simulink model "commhdlQPSKTxRxLoopback"  (R2025b)
settings: Solver=FixedStepDiscrete  StartTime=0.0  StopTime=stopTime  RelTol=1e-3
PostLoadFcn:
  | hScopeConfig = get_param([gcs '/Receiver/QPSK Rx/Frequency and Time Synchronizer/Symbol Synchronizer/No HDL/QPSK Receiver Eye Diagram'],'ScopeConfiguration');
  | 
  | hScopeConfig.OpenAtSimulationStart = false;
  | hScopeConfig.Visible = false;
  | SamplesPerSymbol = 4;
  | %UpsamplesRx = 1;
  | clear hScopeConfig
InitFcn:
  | commhdlQPSKTxRxModelInit;
  | % Rate bridge: ADRV9002/Jupiter radio runs at 15.36 MHz = 2x the 7.68 MHz
  | % (4 samples/symbol @ Rsym=1.92 MHz) the QPSK Rx requires. The deployed
  | % Receiver must downsample the ADC stream by 2. UpsamplesRx=1 fed the QPSK
  | % Rx 8 sps (2x-upsampled) and broke symbol sync / the loopback bit check.
  | UpsamplesRx = 1;   %% T8 RATE FIX: rail 15.36e6 == ADC bus rate,
  | %% no ingress decimation (was 2 when the rail sat on the 7.68e6 rung)
  | UpsamplesTx = 1;
  | clear simTimingOffset;
StopFcn:
  | if exist('simTimingOffset','var')
  |   disp('Simulation completed');
  |   %QPSKTxRxVerification;
  | end
values from neighbouring files (symbols this model uses):
  Config = commhdlQPSKTxRxParameters    [commhdlQPSKTxRxModelInit.m]
  Rsym = eval(get_param(qpskFindTxInputData(gcs),'Rsym'))    [commhdlQPSKTxRxModelInit.m]
undefined symbols (not defined in the file or in its folder): Add, fsym, randsrc, RandStream, Shift
libraries: hdlsllib x143, simulink x45, dspsigops x34, dsphdlfiltering2 x6, dsphdlsigops2 x4, dsphdlmathfun2 x4, commdigbbndpm3 x4, dspmlti4 x2, commchan3 x1, commrflib2 x1, commcnvcod2 x1
(part 8 of 8)

== matlab function commhdlQPSKTxRxLoopback/TxRxComposite/CanaryFast ==
  data: x input; f2 output; f3 output; f4 output; f5 output
function [f2,f3,f4,f5] = canaryFast(x)
%#codegen
persistent r2 r3 r4 r5
if isempty(r2), r2=uint32(0); r3=uint32(0); r4=uint32(0); r5=uint32(0); end
f2=r2; f3=r3; f4=r4; f5=r5;
a = stg(x, uint32(2654435761), uint32(2166136261));
b = stg(a, uint32(2246822519), uint32(3266489917));
c = stg(b, uint32(3299170593), uint32(668265263));
d = stg(c, uint32(374761393),  uint32(2542024007));
e = stg(d, uint32(2869860233), uint32(1540483477));
r2 = b;
r3 = c;
r4 = d;
r5 = e;
end
function y = stg(x, K, C)
y = bitxor(uint32(bitand(bitshift(uint64(x) * uint64(K), -13), uint64(4294967295))), C);
end

== matlab function commhdlQPSKTxRxLoopback/TxRxComposite/CanaryRef ==
  data: x input; r2 output; r3 output; r4 output; r5 output
function [r2,r3,r4,r5] = canaryRef(x)
%#codegen
persistent m2 m3 m4 m5
if isempty(m2), m2=uint32(0); m3=uint32(0); m4=uint32(0); m5=uint32(0); end
% second halves (computed on last beat's midpoints) -- outputs match
% CanaryFast's registered outputs beat-for-beat
r2 = stg(m2, uint32(2246822519), uint32(3266489917));
c  = stg(m3, uint32(3299170593), uint32(668265263));
r3 = c;
d  = stg(stg(m4, uint32(3299170593), uint32(668265263)), uint32(374761393), uint32(2542024007));
r4 = d;
e3 = stg(stg(m5, uint32(3299170593), uint32(668265263)), uint32(374761393), uint32(2542024007));
r5 = stg(e3, uint32(2869860233), uint32(1540483477));
% first halves for NEXT beat
a = stg(x, uint32(2654435761), uint32(2166136261));
b = stg(a, uint32(2246822519), uint32(3266489917));
m2 = a;
m3 = b;
m4 = b;
m5 = b;
end
function y = stg(x, K, C)
y = bitxor(uint32(bitand(bitshift(uint64(x) * uint64(K), -13), uint64(4294967295))), C);
end

== matlab function commhdlQPSKTxRxLoopback/TxRxComposite/CanaryScore ==
  data: f2 input; y output; f3 input; f4 input; f5 input; r2 input; r3 input; r4 input; r5 input
function y = canaryScore(f2,f3,f4,f5,r2,r3,r4,r5)
%#codegen
persistent c2 c3 c4 c5 warm
if isempty(c2), c2=uint8(0); c3=uint8(0); c4=uint8(0); c5=uint8(0); warm=uint8(0); end
if warm < uint8(8)
  warm = warm + uint8(1);
else
  if f2 ~= r2 && c2 < uint8(255), c2 = c2 + uint8(1); end
  if f3 ~= r3 && c3 < uint8(255), c3 = c3 + uint8(1); end
  if f4 ~= r4 && c4 < uint8(255), c4 = c4 + uint8(1); end
  if f5 ~= r5 && c5 < uint8(255), c5 = c5 + uint8(1); end
end
y = bitor(bitor(uint32(c2), bitshift(uint32(c3),8)), ...
          bitor(bitshift(uint32(c4),16), bitshift(uint32(c5),24)));

== matlab function commhdlQPSKTxRxLoopback/Transmitter/QPSK Tx/Bit Packetizer/Data Bits FIFO/MATLAB Function1 ==
  data: wr input; full output; rd input; dataBitsPerPacket parameter
function full = fcn(wr,rd,dataBitsPerPacket)
%#codegen
     
    depth = dataBitsPerPacket*2 - 1;
    persistent count;
    if isempty(count)
        count = fi(0,0,nextpow2(depth),0,hdlfimath);
    end

    if wr
        count(:) = count + 1;
    end
    if rd
        count(:) = count - 1;
    end

    full = (count > depth);

end

== matlab function commhdlQPSKTxRxLoopback/TxRxComposite/Receiver/QPSK Rx/Frequency and Time Synchronizer/Symbol Synchronizer/Interpolation Control Shadow ==
  data: Delta input; mu output; Underflow output
function [mu,Underflow] = Interpolation_ctrl(Delta)
% Implementation of modulo-1 counter for interpolation control listed in
% Figure 8.4.19 of "Digital Communications - A Discrete-Time Approach"
% by Michael Rice. See design details in Chapter 8.4.3 of the same book.
% 
% Input:
%   Delta - Loop filter output. If loop is in lock, delta would be small
% Output:
%   Underflow - Indicator of counter underflow. This is the strobe signal
%               for downstream processing
%   mu - Difference between actual sampling instant and the optimal instant,
%        between zero and one
%#codegen

% countReg - Counter value delayed by 1 sample
% muReg - The estimated timing error normalized by half QPSK symbols

   mask = fi(1-2^(-10),1,11,10);
   
   persistent countReg underflowReg muReg;
   if isempty(countReg)
       countReg  = fi(0.125,1,11,10); %% shadow leading-beat offset compensation
       muReg = fi(0,1,11,10);
       underflowReg = false;
   end
   
   
   Underflow = underflowReg;
   mu = muReg;   
   
   
      % T8.4 anti-wedge clamp: if Delta <= -0.125 the decrementing counter
   % never underflows (strobes stop FOREVER -- Class-4 wedge / Class-1
   % episode mechanism; see tb_timing_wedge.v). Bound Delta so the
   % counter always decrements by >= 1 LSB.
   wlim = fi(127/1024,1,11,10);
   if Delta > wlim
       Delta = wlim;
   elseif Delta < -wlim
       Delta = fi(-127/1024,1,11,10);
   end
   counter = bitand(mask,countReg)-Delta-fi(0.125,1,11,10); % decrementing counter
   
   % if countReg is a nonnegative number,
   % then mod(countReg,1) equals the fractional part of countReg
   if counter < 0
       underflowReg = true;
       muReg = bitshift(bitand(mask,countReg),3);
       countReg = fi(counter+1,1,11,10);% create underflow to counter
   else
       underflowReg = false;
       countReg = fi(counter,1,11,10);
   end
   


end

== matlab function commhdlQPSKTxRxLoopback/TxRxComposite/Receiver/QPSK Rx/Frequency and Time Synchronizer/Symbol Synchronizer/ShadowScoreIC ==
  data: muP input; divBeat output; muS input; undP input; undS input; divCnt output
function [divBeat, divCnt] = shadowScoreIC(muP, muS, undP, undS)
%#codegen
persistent db dc bt mPrev
if isempty(db), db=uint32(0); dc=uint32(0); bt=uint32(0); mPrev=false; end
bt = bt + uint32(1);
m = (muP ~= muS) || (undP ~= undS);
if m && ~mPrev
  if db == uint32(0), db = bt; end
  if dc < uint32(4294967295), dc = dc + uint32(1); end
end
mPrev = m;
divBeat = db; divCnt = dc;

== matlab function commhdlQPSKTxRxLoopback/TxRxComposite/Receiver/QPSK Rx/Frequency and Time Synchronizer/Carrier Synchronizer/ShadowScoreCS ==
  data: pP input; divBeat output; pS input; iP input; iS input; divCnt output
function [divBeat, divCnt] = shadowScoreCS(pP, pS, iP, iS)
%#codegen
persistent db dc bt mPrev
if isempty(db), db=uint32(0); dc=uint32(0); bt=uint32(0); mPrev=false; end
bt = bt + uint32(1);
m = (pP ~= pS) || (iP ~= iS);
if m && ~mPrev
  if db == uint32(0), db = bt; end
  if dc < uint32(4294967295), dc = dc + uint32(1); end
end
mPrev = m;
divBeat = db; divCnt = dc;

== matlab function commhdlQPSKTxRxLoopback/TxRxComposite/Receiver/QPSK Rx/TelemetrySerializer ==
  data: ssI input fixdt(1,30,23); telI output fixdt(1,16,0); ssP input fixdt(1,30,23); ssD4 input fixdt(1,30,23); ssD6 input fixdt(1,30,23); ssD3 input fixdt(1,30,23); ssD5 input fixdt(1,30,23); ssD2 input fixdt(1,40,24); icW input uint32; csP input fixdt(1,29,29); csI input fixdt(1,39,39); csD7 input fixdt(1,13,10); csD5 input fixdt(1,13,10); csD6 input fixdt(1,29,26); csD2 input fixdt(1,29,29); csD1 input fixdt(1,29,26); csD3 input fixdt(1,39,39); agcI input fixdt(1,34,28); telQ output fixdt(1,16,0)
function [telI, telQ] = telemetrySerializer(ssI, ssP, ssD4, ssD6, ssD3, ssD5, ssD2, icW, ...
    csP, csI, csD7, csD5, csD6, csD2, csD1, csD3, agcI)
%#codegen
persistent slot img
if isempty(slot), slot = uint8(0); img = uint32(0); end
w = uint32(0);
switch slot
  case uint8(0),  w = uint32(reinterpretcast(ssI,  numerictype(0,30,0)));
  case uint8(1),  w = uint32(reinterpretcast(ssP,  numerictype(0,30,0)));
  case uint8(2),  w = uint32(reinterpretcast(ssD4, numerictype(0,30,0)));
  case uint8(3),  w = uint32(reinterpretcast(ssD6, numerictype(0,30,0)));
  case uint8(4),  w = uint32(reinterpretcast(ssD3, numerictype(0,30,0)));
  case uint8(5),  w = uint32(reinterpretcast(ssD5, numerictype(0,30,0)));
  case uint8(6),  w = uint32(bitsliceget(reinterpretcast(ssD2, numerictype(0,40,0)), 32, 1));
  case uint8(7),  w = uint32(bitsliceget(reinterpretcast(ssD2, numerictype(0,40,0)), 40, 33));
  case uint8(8),  w = icW;
  case uint8(9),  w = uint32(reinterpretcast(csP, numerictype(0,29,0)));
  case uint8(10), w = uint32(bitsliceget(reinterpretcast(csI, numerictype(0,39,0)), 32, 1));
  case uint8(11), w = uint32(bitsliceget(reinterpretcast(csI, numerictype(0,39,0)), 39, 33));
  case uint8(12), w = bitor(uint32(reinterpretcast(csD7, numerictype(0,13,0))), ...
                      bitshift(uint32(reinterpretcast(csD5, numerictype(0,13,0))), 13));
  case uint8(13), w = uint32(reinterpretcast(csD6, numerictype(0,29,0)));
  case uint8(14), w = uint32(reinterpretcast(csD2, numerictype(0,29,0)));
  case uint8(15), w = uint32(reinterpretcast(csD1, numerictype(0,29,0)));
  case uint8(16), w = uint32(bitsliceget(reinterpretcast(csD3, numerictype(0,39,0)), 32, 1));
  case uint8(17), w = uint32(bitsliceget(reinterpretcast(csD3, numerictype(0,39,0)), 39, 33));
  case uint8(18), w = uint32(bitsliceget(reinterpretcast(real(agcI), numerictype(0,34,0)), 32, 1));
  case uint8(19), w = uint32(bitsliceget(reinterpretcast(real(agcI), numerictype(0,34,0)), 34, 33));
  case uint8(20), w = uint32(bitsliceget(reinterpretcast(imag(agcI), numerictype(0,34,0)), 32, 1));
  case uint8(21), w = uint32(bitsliceget(reinterpretcast(imag(agcI), numerictype(0,34,0)), 34, 33));
  case uint8(22), w = uint32(2781216750);
  otherwise,      w = img;
end
slot = slot + uint8(1);
if slot >= uint8(24)
  slot = uint8(0);
  img = img + uint32(1);
end
telI = reinterpretcast(uint16(bitshift(w, -16)), numerictype(1,16,0));
telQ = reinterpretcast(uint16(bitand(w, uint32(65535))), numerictype(1,16,0));

== matlab function commhdlQPSKTxRxLoopback/TxRxComposite/Transmitter/Input Data/ByteBitShifter ==
  data: enable input; bit output; reset input; start input; extWord input; extWordAvail input; extWordFirst input; popToggle output
function [bit, popToggle] = byteBitShifterBlk(enable, reset, start, extWord, extWordAvail, extWordFirst)
% Block wrapper around qpskByteBitShifter (the unit-tested single source
% of truth). Persistent state only; the effective enable matches the
% Message Generator chart's active condition (enable && ~reset) so the
% shifter emits bits on exactly the generator's bit steps. pop is
% exported as a toggle (one flip per word latch OR discard) to survive
% the slow->fast rate crossing; upstream edge-detects it into a pulse.
persistent state tog
if isempty(state)
    state = qpskByteBitShifter();
    tog = false;
end
en = logical(enable) && ~logical(reset);
[bit, pop, state] = qpskByteBitShifter(state, en, logical(start), ...
    uint64(extWord), logical(extWordAvail), logical(extWordFirst));
if pop
    tog = ~tog;
end
popToggle = tog;

== matlab function commhdlQPSKTxRxLoopback/TxRxComposite/Transmitter/Input Data/FEC Tx Encoder K5/TxGateK5 ==
  data: bitIn input; infoBit output; enable input; reset input; start input; encReset output; infoValid output; beatIdx output; frameValid output; frameStart output
function [infoBit, encReset, infoValid, beatIdx, frameValid, frameStart] = fecTxGateK5(bitIn, enable, reset, start)
%#codegen
% sync-semantics (RXROOT E11c): locals in, outputs from locals, persist last.
persistent beat armed;
INFO=uint16(1084); NIN=uint16(1088); PAYLOAD=uint16(2240);
if isempty(beat), beat=uint16(0); armed=false; end
b=beat; a=armed;
infoBit=false; encReset=false; infoValid=false; beatIdx=uint16(0);
frameValid=false; frameStart=false;
en = logical(enable) && ~logical(reset);
if en
  if start, b=uint16(0); a=true; encReset=true; end
  if a
    if b < INFO
      infoBit = logical(bitIn); infoValid = true;
    elseif b < NIN
      infoBit = false;          infoValid = true;   % K-1 zero tail flush
    end
    beatIdx = b; frameValid = true; frameStart = (b==uint16(0));
    if b < PAYLOAD-uint16(1), b=b+uint16(1); else, b=uint16(0); end
  end
end
beat=b; armed=a;

== matlab function commhdlQPSKTxRxLoopback/TxRxComposite/Transmitter/Input Data/FEC Tx Encoder K5/ConvEncK5 ==
  data: infoBit input; codedPair output; encReset input; infoValid input
function codedPair = fecConvEncK5(infoBit, encReset, infoValid)
%#codegen
persistent sr;
if isempty(sr), sr = false(1,4); end
srUse = sr;
if encReset, srUse = false(1,4); end   % reset-then-advance (zero frame state)
in = logical(infoBit);
s0=in; s1=srUse(1); s2=srUse(2); s3=srUse(3); s4=srUse(4);
g0 = xor(s0, xor(s1, xor(s2, s4)));   % poly 35 oct = 11101
g1 = xor(s0, xor(s3, s4));            % poly 23 oct = 10011
codedPair = [g0; g1];
% state update: advance ONLY on infoValid, else HOLD (anti-zero-stuff gate)
if infoValid
  sr = [in, srUse(1:3)];
else
  sr = srUse;
end

== matlab function commhdlQPSKTxRxLoopback/Transmitter/QPSK Tx/Bit Packetizer/Data Bits FIFO/RAM Frame Status Indicator ==
  data: push input; out output; pop input; dataBitsPerPacket parameter
function out = fcn(push,pop,dataBitsPerPacket)

   persistent pushCount popCount frameCount;
   if isempty(pushCount)
       pushCount = fi(0,0,nextpow2(dataBitsPerPacket),0,hdlfimath);
       frameCount = fi(0,0,2,0,hdlfimath);
       popCount = fi(0,0,nextpow2(dataBitsPerPacket),0,hdlfimath);
   end
   
   if (pushCount == dataBitsPerPacket-1) && push
       frameCount(:) = frameCount + 1;
   end
   if (popCount == dataBitsPerPacket-1) && pop
       frameCount(:) = frameCount - 1;
   end

   if push
       if pushCount == dataBitsPerPacket - 1
           pushCount(:) = 0;
       else
           pushCount(:) = pushCount + 1;
       end
   end

   if pop 
       if popCount == dataBitsPerPacket - 1
           popCount(:) = 0;
       else
           popCount(:) = popCount + 1;
       end
   end

   out = frameCount;

end

== matlab function commhdlQPSKTxRxLoopback/TxRxComposite/Transmitter/Input Data/FEC Tx Encoder K5/TxInterleaveK5 ==
  data: codedPair input; dataOut output; infoValid input; beatIdx input; frameValid input; frameStart input
function dataOut = fecTxInterleaveK5(codedPair, infoValid, beatIdx, frameValid, frameStart)
%#codegen
persistent ramA ramB rdBank wptr rrow rcol;
CODED=uint16(2176); COLS=uint16(16); ROWS=uint16(136);
FILL = logical([1 1 1 1 1 1 1 1 1 0 0 0 0 0 1 1 1 1 0 1 1 1 1 1 0 0 0 1 0 1 1 1 0 0 1 1 0 0 1 0 0 0 0 0 1 0 0 1 0 1 0 0 1 1 1 0 1 1 0 1 0 0 0 1]);   % 64-bit PN9 filler (T8 fix 6bcaa62)
if isempty(ramA), ramA=false(1,2176); ramB=false(1,2176); rdBank=false; wptr=uint16(0); rrow=uint16(0); rcol=uint16(0); end
rb=rdBank; w=wptr; rr=rrow; cc=rcol;
dataOut=false;
wr0=uint16(0); wr1=uint16(0); v0=false; v1=false; doW0=false; doW1=false;
if frameValid
  if frameStart, w=uint16(0); rb=~rb; end
  % ---- READ side (previous frame, opposite bank), legacy perm r*COLS+c ----
  % divisionless read address: rr (row 0..ROWS-1) / cc (col 0..COLS-1) are
  % incremental counters, reset on beatIdx==0, advancing +1 row with col carry
  % per in-range beat -- replaces the old per-beat divide-by-ROWS. No divide.
  if beatIdx < CODED
    % precondition: bit-exactness requires a contiguous beatIdx hitting 0 once per
    % frame to re-seed the row/col counters (the old stateless per-beat address
    % arithmetic derived the address from beatIdx alone and needed no such reset).
    if beatIdx == 0, rr = uint16(0); cc = uint16(0); end
    perm = rr*COLS + cc;
    if perm < CODED
      if rb, dataOut = ramB(double(perm)+1); else, dataOut = ramA(double(perm)+1); end
    end
    rr = rr + uint16(1);
    if rr == ROWS, rr = uint16(0); cc = cc + uint16(1); end
  else
    dataOut = FILL(double(beatIdx-CODED)+1);   % PN9 filler, beats CODED..2239
  end
  % ---- WRITE side: two coded bits per encoder-advance beat ----
  if infoValid
    if w < CODED, wr0=w; v0=(codedPair(1)~=0); doW0=true; w=w+uint16(1); end
    if w < CODED, wr1=w; v1=(codedPair(2)~=0); doW1=true; w=w+uint16(1); end
  end
end
% ---- persist state last (write bank = opposite of read bank) ----
if doW0
  if rb, ramA(double(wr0)+1)=v0; else, ramB(double(wr0)+1)=v0; end
end
if doW1
  if rb, ramA(double(wr1)+1)=v1; else, ramB(double(wr1)+1)=v1; end
end
rdBank=rb; wptr=w; rrow=rr; rcol=cc;

== matlab function commhdlQPSKTxRxLoopback/TxRxComposite/ByteWordBuffer ==
  data: dataIn input; word output; validIn input; popReq input; firstIn input; avail output; readyNext output; wordFirst output
function [word, avail, readyNext, wordFirst] = byteWordBufferBlk(dataIn, validIn, popReq, firstIn)
% Block wrapper around qpskByteWordBuffer (unit-tested single source of
% truth); persistent state only. readyNext = the post-update registered
% ready; an external Delay (IC=1) turns it back into the AXIS tready.
% firstIn/wordFirst carry the in-band first-word marker alongside data.
persistent state
if isempty(state)
    state = qpskByteWordBuffer();
end
[word, avail, ~, wordFirst, state] = qpskByteWordBuffer(state, uint64(dataIn), ...
    logical(validIn), logical(popReq), logical(firstIn));
readyNext = state.readyReg;

== matlab function commhdlQPSKTxRxLoopback/TxRxComposite/ByteSerializer ==
  data: bitIn input; word output; bitValid input; start input; ready input; wordTog output; wordLast output; wordFirst output
function [word, wordTog, wordLast, wordFirst] = byteSerializerBlk(bitIn, bitValid, start, ready)
% Block wrapper around qpskByteSerializer (unit-tested single source of
% truth); persistent state only. word/wordLast are HELD stable between
% emissions; wordTog flips once per emitted word so the slow->fast rate
% crossing cannot drop or repeat it -- the 30.72M BeatGate edge-detects
% it into exactly one accepted AXIS beat. Dropped words (ready low at
% completion) do not toggle: drop means NO beat, never a stall.
% K5 kit: 16 words/frame = the first 64*16 of
% the 1084 decoded info bits; the trailing 60 are dropped by start-reset.
persistent state tog heldWord heldLast heldFirst firstNext
if isempty(state)
    state = qpskByteSerializer();
    tog = false; heldWord = uint64(0); heldLast = false;
    heldFirst = true; firstNext = true;
end
% presentation is decoupled from acceptance (ADI S2MM source style):
% the offered beat must refresh on EVERY completed word or the DMA's
% SYNC_TRANSFER_START gate can wait forever on a frozen user flag /
% accept a stale word. ready at the pin only decides acceptance, so
% the core serializer runs with ready=true and unaccepted beats are
% simply superseded.
[w, wv, wl, ~, state] = qpskByteSerializer(state, logical(bitIn), ...
    logical(bitValid), logical(start), true, uint16(16));
if wv
    heldWord = w; heldLast = logical(wl); tog = ~tog;
    heldFirst = firstNext; firstNext = logical(wl);
end
word = heldWord; wordTog = tog; wordLast = heldLast; wordFirst = heldFirst;

== matlab function commhdlQPSKTxRxLoopback/TxRxComposite/ByteRxFifo ==
  data: word input uint64; outWord output uint64; tog input boolean; wLast input boolean; wFirst input boolean; ready input boolean; valid output boolean; outLast output boolean; outFirst output boolean; ovf output uint32
function [outWord, valid, outLast, outFirst, ovf] = byteRxFifo(word, tog, wLast, wFirst, ready)
%#codegen
% 64-deep elastic FIFO: enqueue on serializer toggle edge, dequeue on
% accepted AXIS beat. Drop-newest + count on full (stall > ~19 ms).
persistent mem memFl wr rd prev ovfCnt
if isempty(wr)
    mem = zeros(64,1,'uint64'); memFl = zeros(64,1,'uint8');
    wr = uint16(0); rd = uint16(0); prev = false; ovfCnt = uint32(0);
end
if logical(tog) ~= prev
    nxt = uint16(mod(uint32(wr) + 1, 64));
    if nxt == rd
        % full: DROP OLDEST (advance rd) so the presented head converges
        % to fresh data when unconsumed -- preserves the DMA start-sync
        % contract (the old supersede semantics) while keeping 64 words
        % of elasticity for transient stalls. Never deadlocks on a
        % mid-frame stale head.
        rd = uint16(mod(uint32(rd) + 1, 64));
        ovfCnt = ovfCnt + uint32(1);
    end
    mem(uint32(wr)+1)   = uint64(word);
    memFl(uint32(wr)+1) = uint8(wLast) + uint8(2)*uint8(wFirst);
    wr = nxt;
end
prev = logical(tog);
valid = (wr ~= rd);
outWord  = mem(uint32(rd)+1);
fl = memFl(uint32(rd)+1);
outLast  = bitand(fl, uint8(1)) ~= uint8(0);
outFirst = bitand(fl, uint8(2)) ~= uint8(0);
if valid && logical(ready)
    rd = uint16(mod(uint32(rd) + 1, 64));
end
ovf = ovfCnt;

== matlab function commhdlQPSKTxRxLoopback/TxRxComposite/Receiver/QPSK Rx/Frequency and Time Synchronizer/Carrier Synchronizer/ValidCensus ==
  data: vin input boolean; cvin output uint32; vlf input boolean; vout input boolean; cvlf output uint32; cvout output uint32
function [cvin, cvlf, cvout] = validCensus(vin, vlf, vout)
%#codegen
persistent a b c
if isempty(a), a = uint32(0); b = uint32(0); c = uint32(0); end
if vin,  a = a + uint32(1); end
if vlf,  b = b + uint32(1); end
if vout, c = c + uint32(1); end
cvin = a; cvlf = b; cvout = c;

== matlab function commhdlQPSKTxRxLoopback/TxRxComposite/ByteCensus ==
  data: v input boolean; cnt output uint32
function cnt = byteCensus(v)
%%#codegen
persistent a
if isempty(a), a = uint32(0); end
if v, a = a + uint32(1); end
cnt = a;

== matlab function commhdlQPSKTxRxLoopback/TxRxComposite/Receiver/QPSK Rx/Frequency and Time Synchronizer/Preamble Detector/PdCensus ==
  data: done input boolean; w1 output uint32; succ input boolean; off input uint16; taSync input boolean; nEnt input uint8; vPop input boolean; w2 output uint32; w3 output uint32
function [w1, w2, w3] = pdCensus(done, succ, off, taSync, nEnt, vPop)
%#codegen
persistent cDone cSucc pSucc cSync cPop hiw offL
if isempty(cDone)
    cDone = uint32(0); cSucc = uint32(0); pSucc = false;
    cSync = uint32(0); cPop = uint32(0); hiw = uint8(0); offL = uint16(0);
end
if done,   cDone = cDone + uint32(1); offL = off; end
if succ && ~pSucc, cSucc = cSucc + uint32(1); end
pSucc = logical(succ);
if taSync, cSync = cSync + uint32(1); end
if vPop,   cPop  = cPop  + uint32(1); end
if nEnt > hiw, hiw = nEnt; end
w1 = bitor(bitshift(bitand(cSync, uint32(65535)), 16), bitand(cDone, uint32(65535)));
w2 = bitor(bitor(bitshift(uint32(hiw), 24), ...
     bitshift(bitand(cSucc, uint32(255)), 16)), uint32(offL));
w3 = cPop;

== matlab function commhdlQPSKTxRxLoopback/TxRxComposite/Receiver/QPSK Rx/Frequency and Time Synchronizer/Packet Controller/PcCensus ==
  data: pend input boolean; w1 output uint32; endp input boolean; startp input boolean; w2 output uint32
function [w1, w2] = pcCensus(pend, endp, startp)
%#codegen
persistent cPend pPend cEnd cStart
if isempty(cPend)
    cPend = uint32(0); pPend = false; cEnd = uint32(0); cStart = uint32(0);
end
if pend && ~pPend, cPend = cPend + uint32(1); end
pPend = logical(pend);
if endp,   cEnd   = cEnd   + uint32(1); end
if startp, cStart = cStart + uint32(1); end
w1 = bitor(bitshift(bitand(cEnd, uint32(65535)), 16), bitand(cStart, uint32(65535)));
w2 = cPend;

== matlab function commhdlQPSKTxRxLoopback/Receiver/QPSK Rx/Frequency and Time Synchronizer/Packet Controller/sample discard controller ==
  data: dataIn input; validIn input; dataOut output; startIn input; endIn input; startOut output; endOut output; validOut output
function [dataOut,startOut,endOut,validOut] = controller(dataIn,validIn,startIn,endIn)
%#codegen

   persistent active dataOutReg validOutReg startOutReg endOutReg;
   if isempty(active)
      active  = false;
      dataOutReg = cast(0,'like',dataIn);
      validOutReg = false;
      startOutReg = false;
      endOutReg = false;
   end
   
   dataOut = dataOutReg;
   validOut = validOutReg;
   startOut = startOutReg;
   endOut = endOutReg;
   
   startOutReg = startIn;
   endOutReg = endIn;
   
   if startIn
       active = true;
   end
   
   if active
       dataOutReg(:) = dataIn;
       validOutReg = validIn;
   else
       dataOutReg(:) = 0;
       validOutReg = false;
   end
   
   if endIn
       if active 
           endOutReg = true;
       else
           endOutReg = false;
       end
       active = false;
   end
end

== matlab function commhdlQPSKTxRxLoopback/TxRxComposite/Receiver/QPSK Rx/Frequency and Time Synchronizer/Phase Ambiguity Estimation and Correction/PaCensus ==
  data: negRe input boolean; w output uint32; negIm input boolean
function w = paCensus(negRe, negIm)
%#codegen
persistent cFlip pSec init
if isempty(cFlip)
    cFlip = uint32(0); pSec = uint8(0); init = false;
end
sec = uint8(2)*uint8(negRe) + uint8(negIm);
if init && sec ~= pSec, cFlip = cFlip + uint32(1); end
pSec = sec; init = true;
w = bitor(bitshift(uint32(sec), 30), bitand(cFlip, uint32(1073741823)));

== matlab function commhdlQPSKTxRxLoopback/TxRxComposite/Receiver/QPSK Rx/Frequency and Time Synchronizer/Preamble Detector/PdTelemetry ==
  data: validIn input boolean; telI output fixdt(1,16,0); dI input int16; dQ input int16; thrEx input boolean; tRef input uint16; tOff input uint16; done input boolean; newPk input boolean; succ input boolean; sync input boolean; armed input boolean; taRef input uint16; accOff input uint16; fifoEnt input uint16; vPop input boolean; tRefLong input uint32; runMax input uint32; heldTs input uint32; telQ output fixdt(1,16,0)
function [telI, telQ] = pdTelemetry(validIn, dI, dQ, thrEx, tRef, tOff, done, newPk, succ, sync, armed, taRef, accOff, fifoEnt, vPop, tRefLong, runMax, heldTs)
%#codegen
persistent slot symCtr beatCnt aDone aNewPk aThrEx aSync aVPop s0 s1 s2 s3 s4 s5 s6
if isempty(slot)
    slot = uint8(7); symCtr = uint32(0); beatCnt = uint8(0);
    aDone = false; aNewPk = false; aThrEx = false; aSync = false; aVPop = false;
    s0 = uint32(0); s1 = uint32(0); s2 = uint32(0); s3 = uint32(0);
    s4 = uint32(0); s5 = uint32(0); s6 = uint32(0);
end
aDone = aDone || done; aNewPk = aNewPk || newPk; aThrEx = aThrEx || thrEx;
aSync = aSync || sync; aVPop = aVPop || vPop;
if beatCnt < uint8(7), beatCnt = beatCnt + uint8(1); end
if validIn
    symCtr = symCtr + uint32(1);
    flags = uint32(aDone) + bitshift(uint32(aNewPk),1) + bitshift(uint32(succ),2) + ...
            bitshift(uint32(aThrEx),3) + bitshift(uint32(aSync),4) + bitshift(uint32(armed),5);
    s0 = bitor(bitor(bitor(bitshift(uint32(14),28), bitshift(uint32(bitand(tRef,uint16(2047))),17)), ...
         bitshift(uint32(bitand(tOff,uint16(2047))),6)), flags);
    s1 = bitor(bitshift(uint32(reinterpretcast(dI,numerictype(0,16,0))),16), ...
         uint32(reinterpretcast(dQ,numerictype(0,16,0))));
    s2 = bitor(bitor(bitor(bitshift(uint32(bitand(taRef,uint16(2047))),21), ...
         bitshift(uint32(bitand(accOff,uint16(2047))),10)), ...
         bitshift(uint32(bitand(fifoEnt,uint16(511))),1)), uint32(aVPop));
    s3 = tRefLong;
    s4 = runMax;
    s5 = heldTs;
    s6 = bitor(bitor(bitshift(uint32(165),24), bitshift(uint32(bitand(uint16(beatCnt),uint16(7))),21)), ...
         bitand(symCtr,uint32(2097151)));
    aDone = false; aNewPk = false; aThrEx = false; aSync = false; aVPop = false;
    beatCnt = uint8(0);
    slot = uint8(0);
end
switch slot
  case uint8(0), w = s0;
  case uint8(1), w = s1;
  case uint8(2), w = s2;
  case uint8(3), w = s3;
  case uint8(4), w = s4;
  case uint8(5), w = s5;
  case uint8(6), w = s6;
  otherwise,     w = uint32(0);
end
if slot < uint8(7), slot = slot + uint8(1); end
telI = reinterpretcast(uint16(bitshift(w, -16)), numerictype(1,16,0));
telQ = reinterpretcast(uint16(bitand(w, uint32(65535))), numerictype(1,16,0));

== matlab function commhdlQPSKTxRxLoopback/TxRxComposite/Receiver/QPSK Rx/Frequency and Time Synchronizer/Preamble Detector/Timing Adjust/P1eArm ==
  data: psTref input; setOut output; psNewpk input; timingOffset input; timingOffsetValid input; accOff input; clrOut output
function [setOut, clrOut] = p1eArm(psTref, psNewpk, timingOffset, timingOffsetValid, accOff)
%#codegen
persistent setR clrR;
if isempty(setR), setR=false; clrR=false; end
setOut = setR; clrOut = clrR;
tr = uint16(psTref); ac = uint16(accOff); to = uint16(timingOffset);
if tr >= ac, d2 = tr - ac; else, d2 = (tr + uint16(1133)) - ac; end
if to >= ac, d1 = to - ac; else, d1 = (to + uint16(1133)) - ac; end
npk = logical(psNewpk); tov = logical(timingOffsetValid);
% v3 qualifier: arm only when the displaced window's fire is provably
% stale (fire at acc + FIFO transit 566 sym precedes the wrap report at
% 1132 -> acc <= 530 with margin).  Late-acc windows are re-anchored by
% the freshest-offset fix already; skipping them is the proven harm case
% (two-capture 6-phase sweeps: acc=454 help 6/6, acc=875 harm 6/6).
% A missed arm falls back to stock behavior (safe).
setR = npk && (d2 == uint16(32)) && (ac <= uint16(530));
clrR = (npk && (d2 ~= uint16(32))) || (tov && (d1 ~= uint16(32)));

== matlab function commhdlQPSKTxRxLoopback/Receiver/QPSK Rx/Frequency and Time Synchronizer/Symbol Synchronizer/Interpolation Control ==
  data: mu output; Delta input; Underflow output
function [mu,Underflow] = Interpolation_ctrl(Delta)
% Implementation of modulo-1 counter for interpolation control listed in
% Figure 8.4.19 of "Digital Communications - A Discrete-Time Approach"
% by Michael Rice. See design details in Chapter 8.4.3 of the same book.
% 
% Input:
%   Delta - Loop filter output. If loop is in lock, delta would be small
% Output:
%   Underflow - Indicator of counter underflow. This is the strobe signal
%               for downstream processing
%   mu - Difference between actual sampling instant and the optimal instant,
%        between zero and one
%#codegen

% countReg - Counter value delayed by 1 sample
% muReg - The estimated timing error normalized by half QPSK symbols

   mask = fi(1-2^(-10),1,11,10);
   
   persistent countReg underflowReg muReg;
   if isempty(countReg)
       countReg  = fi(0,1,11,10);
       muReg = fi(0,1,11,10);
       underflowReg = false;
   end
   
   
   Underflow = underflowReg;
   mu = muReg;   
   
   
      % T8.4 anti-wedge clamp: if Delta <= -0.125 the decrementing counter
   % never underflows (strobes stop FOREVER -- Class-4 wedge / Class-1
   % episode mechanism; see tb_timing_wedge.v). Bound Delta so the
   % counter always decrements by >= 1 LSB.
   wlim = fi(127/1024,1,11,10);
   if Delta > wlim
       Delta = wlim;
   elseif Delta < -wlim
       Delta = fi(-127/1024,1,11,10);
   end
   counter = bitand(mask,countReg)-Delta-fi(0.125,1,11,10); % decrementing counter
   
   % if countReg is a nonnegative number,
   % then mod(countReg,1) equals the fractional part of countReg
   if counter < 0
       underflowReg = true;
       muReg = bitshift(bitand(mask,countReg),3);
       countReg = fi(counter+1,1,11,10);% create underflow to counter
   else
       underflowReg = false;
       countReg = fi(counter,1,11,10);
   end
   


end

== matlab function commhdlQPSKTxRxLoopback/Receiver/QPSK Rx/Frequency and Time Synchronizer/Preamble Detector/Correlator/ThresholdLimiter ==
  settings: fimath=hdlfimath
  data: x input; y output
function y = applyLowerLimit(x)
    % Apply a lower limit to the threshold.
    %#codegen
    
    % Threshold is computed by summing across 63 samples.
    % Set lower limit to be equivalent of all 63 samples
    % having their LSB set to 1 and all others set to 0. 
    lowerLimit = cast(0.01, 'like', x);
    
    if x < lowerLimit
        y = lowerLimit;
    else
        y = x;
    end
end

== matlab function commhdlQPSKTxRxLoopback/Transmitter/Input Data/Message Generator/MATLAB Function ==
  data: enable input; reset input; out output; start output; stop output; valid output; count_out output; msg_count_out output
function [out, start, stop, valid, count_out, msg_count_out] = msggen(enable, reset)

persistent indexCount;
persistent toggle;
persistent msgCount;
persistent msgCountAll;
persistent msgCountBitIndex;

if isempty(indexCount) || isempty(toggle) || isempty(msgCount) || isempty(msgCountBitIndex) || isempty(msgCountAll)
    indexCount = uint32(0);
    msgCount = uint32(1);
    msgCountAll = uint32(1);
    msgCountBitIndex = uint8(0);
    toggle = false;
end

%% Constants
strAscii = dec2bin('ADI Hello World', 8);
msgarray = reshape(strAscii', [1, numel(strAscii)]);
msgbits = logical(msgarray - 48);
msgbitsLen = length(msgbits);

fullMessageLen = uint32(2240-1); % Need the -1 to eat the feedback delay

% Bit counter
% N = 8;% 8-bit counter
% mask = uint32(2^N - 1);
% for k = 1:300
%     msgCount = bitand(msgCount + uint32(1), mask);   % wraps 255 -> 0
% end

%% Logic
if enable && ~reset
    % Set out data
    if indexCount < msgbitsLen % Insert msg
        out = msgbits(indexCount + 1);
        msgCountBitIndex = uint8(0);
    else % Zero padding: varying filler (counter digit + toggle bits)
        % caused periodic false-lock error bursts in the deployed BIST;
        % zero-padded payload matches the verified host golden structure.
        out = false;
        msgCountBitIndex = uint8(0);
    end

    % Flags
    start = indexCount == uint32(0);
    stop = indexCount == fullMessageLen;
    valid = true;

    % Counters
    if fullMessageLen == indexCount
        if msgCount >= 9
            msgCount = uint32(1);
        else
            msgCount = msgCount +  1;
            msgCountAll = msgCountAll + 1;
        end
    end
    if indexCount <= fullMessageLen
        indexCount = indexCount + 1;
    end

else % Enable == false

    if reset
        indexCount = uint32(0);
        % msgCount = uint32(0);
        msgCountBitIndex = uint8(0);
        toggle = false;
    end
    out = false;
    start = false;
    stop = false;
    valid = false;
end

if isempty(indexCount)
    count_out = uint32(0);
else
    count_out = indexCount;
end

msg_count_out = msgCountAll;
